simulink model "tools"  (R2019b)
settings: Solver=VariableStepAuto  StartTime=0.0  StopTime=10.0  RelTol=1e-3
undefined symbols (not defined in the file): pelvisPosition, pelvisVelocity, X, Y, Z
libraries: sm_lib x20, nesl_utility x13, ComponentLibrary x2
settings Model: Creator=hanli  LastModifiedBy=hanli

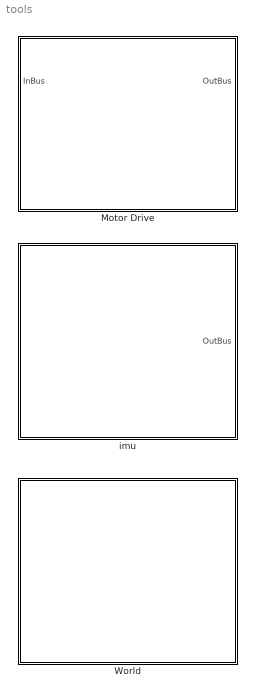
== system tools ==
  Motor Drive : Subsystem  AncestorBlock=ComponentLibrary/Simulation/Elmo Drive  mask{gearRatio=25, rotorInertia=0.000061, encoderResolution=2^13, peakTorque=4.5, peakSpeed=2900*(2*pi/60), initialPosition=0, initialVelocity=0}
      mask prompts: gearRatio "Gear Ratio:"; rotorInertia "Motor rotor inertia (kg*m^2):"; encoderResolution "Input Encoder Resolution (ticks/rev):"; peakTorque "Peak torque of motor (N*m):"; peakSpeed "Peak speed of motor (rad/s):"; initialPosition "Initial Position (rad):"; initialVelocity "Initial Velocity (rad/s):"
      mask Display: image('motor2.JPG'); % Use "Edit Image" on toolstrip to change.
  World : Subsystem  AncestorBlock=ComponentLibrary/Simulation/World
  imu : Subsystem  AncestorBlock=ComponentLibrary/Simulation/VectorNav  mask{preRotationMatrix=eye(3), postRotationMatrix=eye(3)}
      mask prompts: preRotationMatrix "Pre Rotation Matrix:"; postRotationMatrix "Post Rotation Matrix"
      mask Display: image('gx5-25.jpg'); % Use "Edit Image" on toolstrip to change.

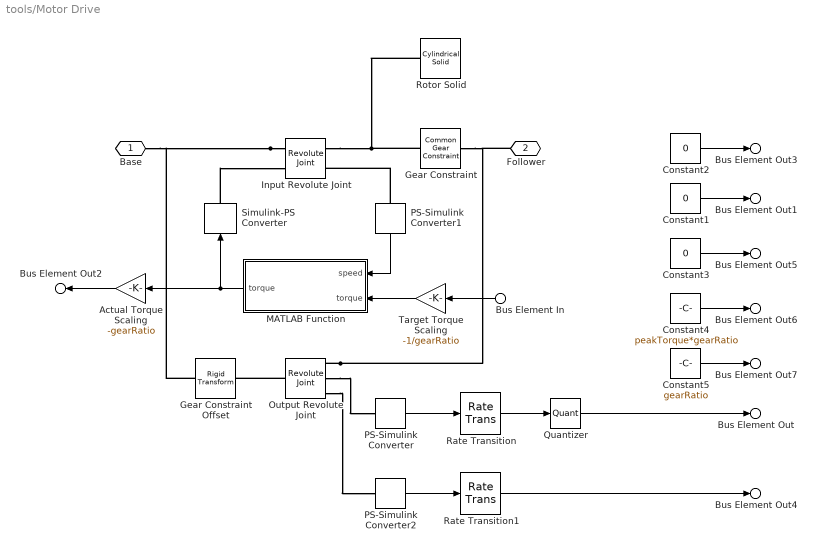
== system tools/Motor Drive ==
  Bus Element In : Inport  PortName=InBus  Element=torque
  Actual Torque Scaling : Gain  Gain=-gearRatio
  Constant1 : Constant  Value=0
  Constant2 : Constant  Value=0  OutDataTypeStr=uint16
  Constant3 : Constant  Value=0
  Constant4 : Constant  Value=peakTorque*gearRatio
  Constant5 : Constant  Value=gearRatio
  Gear Constraint : sm_lib/Gears and Couplings/Gears/Common Gear Constraint  GearType=External  SpecificationType=CenterDistanceRatio  CenterDistance=1e-6  CenterDistanceUnits=m  GearRatio=gearRatio  BaseGearRadius=10.0  BaseGearRadiusUnits=cm  FollGearRadius=10.0  FollGearRadiusUnits=cm  AssemblyGearRotation=Free
      settings: SourceProductName=Simscape Multibody  SourceProductBaseCode=MS
  Gear Constraint Offset : sm_lib/Frames and Transforms/Rigid Transform  TranslationMethod=StandardAxis  TranslationStandardOffset=1e-6  TranslationLengthUnit=m  TranslationStandardAxis=+Y  TranslationCartesianOffset=[0 0 0]  TranslationROffset=0  TranslationROffsetUnits=m  TranslationZOffset=0  TranslationZOffsetUnits=m  TranslationThetaOffset=0  TranslationThetaOffsetUnits=deg  RotationMethod=None  RotationAngleUnits=deg  RotationStandardAxis=+Z  RotationAngle=0.0  RotationArbitraryAxis=[0 0 1]  FollAlignAxisA=+X  BaseAlignAxisA=+Y  FollAlignAxisB=+Y  BaseAlignAxisB=+Z  RotationSequenceAxes=FollowerAxes  RotationSequence=XYX  RotationSequenceAngles=[0 0 0]  RotationSequenceAnglesUnits=deg  RotationMatrix=[1 0 0; 0 1 0; 0 0 1]
  Input Revolute Joint : sm_lib/Joints/Revolute Joint  JointMode=Normal  SenseConstraintForce=off  SenseConstraintForceX=off  SenseConstraintForceY=off  SenseConstraintForceZ=off  SenseConstraintTorque=off  SenseConstraintTorqueX=off  SenseConstraintTorqueY=off  SenseConstraintTorqueZ=off  SenseTotalForce=off  SenseTotalForceX=off  SenseTotalForceY=off  SenseTotalForceZ=off  SenseTotalTorque=off  SenseTotalTorqueX=off  SenseTotalTorqueY=off  SenseTotalTorqueZ=off  CompositeWrenchDir=FollowerOnBase  CompositeWrenchFrame=BaseFrame  EquilibriumPosition=0  EquilibriumPositionUnits=rad  SpringStiffness=0  SpringStiffnessUnits=N*m/rad  DampingCoefficient=0  DampingCoefficientUnits=N*m/(rad/s)  TorqueActuationMode=InputTorque  MotionActuationMode=ComputedMotion  SensePosition=off  SenseVelocity=on  SenseAcceleration=off  SenseTorqueForce=off  SenseLowerLimitTorqueForce=off  SenseUpperLimitTorqueForce=off  LowerLimitSpecify=off  LowerLimitBound=-90  LowerLimitBoundUnits=deg  LowerLimitStiffness=1e4  LowerLimitStiffnessUnits=N*m/deg  LowerLimitDamping=10  LowerLimitDampingUnits=N*m/(deg/s)  LowerLimitTransitionRegionWidth=0.1  LowerLimitTransitionRegionWidthUnits=deg  UpperLimitSpecify=off  UpperLimitBound=90  UpperLimitBoundUnits=deg  UpperLimitStiffness=1e4  UpperLimitStiffnessUnits=N*m/deg  UpperLimitDamping=10  UpperLimitDampingUnits=N*m/(deg/s)  UpperLimitTransitionRegionWidth=0.1  UpperLimitTransitionRegionWidthUnits=deg  PositionTargetSpecify=off  PositionTargetPriority=High  PositionTargetValue=0  PositionTargetValueUnits=deg  VelocityTargetSpecify=off  VelocityTargetPriority=High  VelocityTargetValue=0  VelocityTargetValueUnits=rad/s
  MATLAB Function : MATLAB Function  TreatAsAtomicUnit=on
  Output Revolute Joint : sm_lib/Joints/Revolute Joint  JointMode=Normal  SenseConstraintForce=off  SenseConstraintForceX=off  SenseConstraintForceY=off  SenseConstraintForceZ=off  SenseConstraintTorque=off  SenseConstraintTorqueX=off  SenseConstraintTorqueY=off  SenseConstraintTorqueZ=off  SenseTotalForce=off  SenseTotalForceX=off  SenseTotalForceY=off  SenseTotalForceZ=off  SenseTotalTorque=off  SenseTotalTorqueX=off  SenseTotalTorqueY=off  SenseTotalTorqueZ=off  CompositeWrenchDir=FollowerOnBase  CompositeWrenchFrame=BaseFrame  EquilibriumPosition=0  EquilibriumPositionUnits=rad  SpringStiffness=0  SpringStiffnessUnits=N*m/rad  DampingCoefficient=1  DampingCoefficientUnits=N*m/(rad/s)  TorqueActuationMode=NoTorque  MotionActuationMode=ComputedMotion  SensePosition=on  SenseVelocity=on  SenseAcceleration=off  SenseTorqueForce=off  SenseLowerLimitTorqueForce=off  SenseUpperLimitTorqueForce=off  LowerLimitSpecify=off  LowerLimitBound=-90  LowerLimitBoundUnits=deg  LowerLimitStiffness=1e4  LowerLimitStiffnessUnits=N*m/deg  LowerLimitDamping=10  LowerLimitDampingUnits=N*m/(deg/s)  LowerLimitTransitionRegionWidth=0.1  LowerLimitTransitionRegionWidthUnits=deg  UpperLimitSpecify=off  UpperLimitBound=90  UpperLimitBoundUnits=deg  UpperLimitStiffness=1e4  UpperLimitStiffnessUnits=N*m/deg  UpperLimitDamping=10  UpperLimitDampingUnits=N*m/(deg/s)  UpperLimitTransitionRegionWidth=0.1  UpperLimitTransitionRegionWidthUnits=deg  PositionTargetSpecify=on  PositionTargetPriority=High  PositionTargetValue=initialPosition  PositionTargetValueUnits=rad  VelocityTargetSpecify=on  VelocityTargetPriority=High  VelocityTargetValue=initialVelocity  VelocityTargetValueUnits=rad/s
  PS-Simulink Converter : nesl_utility/PS-Simulink Converter  PhysicalDomain=network_engine_domain  SubClassName=ps_output  LeftPortType=input  RightPortType=output  PseudoPeriodic=off  Frequencies=[]  Unit=rad  AffineConversion=off
  PS-Simulink Converter1 : nesl_utility/PS-Simulink Converter  PhysicalDomain=network_engine_domain  SubClassName=ps_output  LeftPortType=input  RightPortType=output  PseudoPeriodic=off  Frequencies=[]  Unit=rad/s  AffineConversion=off
  PS-Simulink Converter2 : nesl_utility/PS-Simulink Converter  PhysicalDomain=network_engine_domain  SubClassName=ps_output  LeftPortType=input  RightPortType=output  PseudoPeriodic=off  Frequencies=[]  Unit=rad/s  AffineConversion=off
  Quantizer : Quantizer  QuantizationInterval=(2*pi)/(encoderResolution*gearRatio)
  Rate Transition : RateTransition  Deterministic=off  InitialCondition=initialPosition  OutPortSampleTimeOpt=Inherit
  Rate Transition1 : RateTransition  Deterministic=off  InitialCondition=initialPosition  OutPortSampleTimeOpt=Inherit
  Rotor Solid : sm_lib/Body Elements/Cylindrical Solid  GraphicAmbientColor=[0.15 0.15 0.15 1.0]  BasedOnType=Density  CenterOfMass=[0; 0; 0]  CenterOfMassUnits=m  GraphicDiffuseColor=[0.5 0.5 0.5]  CylinderLength=1  CylinderLengthUnits=m  CylinderRadius=1  CylinderRadiusUnits=m  Density=1000  DensityUnits=kg/m^3  DoExposeReferenceFrame=on  GraphicEmissiveColor=[0.0 0.0 0.0 1.0]  ExportEntireGeometry=off  SerializedFrames=<Frames/>  MarkerShape=Sphere  MarkerSize=10  GraphicType=None  InertiaType=Custom  Mass=0  MassUnits=kg  MomentsOfInertia=[0; 0; rotorInertia]  MomentsOfInertiaUnits=kg*m^2  GraphicOpacity=1.0  ProductsOfInertia=[0; 0; 0]  ProductsOfInertiaUnits=kg*m^2  GraphicShininess=75  GraphicSpecularColor=[0.5 0.5 0.5 1.0]  GraphicVisPropType=SimpleVisualProperties
  Simulink-PS Converter : nesl_utility/Simulink-PS Converter  PhysicalDomain=network_engine_domain  SubClassName=ps_input  LeftPortType=input  RightPortType=output  PseudoPeriodic=off  Frequencies=[]  NoiseDistribution=none  NoiseParameters=[]  Unit=N*m  AffineConversion=off  FilteringAndDerivatives=zero  SimscapeFilterOrder=1  InputFilterTimeConstant=0.001  UdotUserProvided=1
  Target Torque Scaling : Gain  Gain=-1/gearRatio
  Base : PMIOPort  Side=Left
  Follower : PMIOPort  Port=2  Side=Right
  Bus Element Out3 : Outport  VectorParamsAs1DForOutWhenUnconnected=off  PortName=OutBus  Element=statusWord
  Bus Element Out : Outport  VectorParamsAs1DForOutWhenUnconnected=off  PortName=OutBus  Element=position
  Bus Element Out4 : Outport  VectorParamsAs1DForOutWhenUnconnected=off  PortName=OutBus  Element=velocity
  Bus Element Out2 : Outport  VectorParamsAs1DForOutWhenUnconnected=off  PortName=OutBus  Element=torque
  Bus Element Out1 : Outport  VectorParamsAs1DForOutWhenUnconnected=off  PortName=OutBus  Element=driveTemperature
  Bus Element Out5 : Outport  VectorParamsAs1DForOutWhenUnconnected=off  PortName=OutBus  Element=dcLinkVoltage
  Bus Element Out6 : Outport  VectorParamsAs1DForOutWhenUnconnected=off  PortName=OutBus  Element=torqueLimit
  Bus Element Out7 : Outport  VectorParamsAs1DForOutWhenUnconnected=off  PortName=OutBus  Element=gearRatio
  wires:
  PS-Simulink Converter2/1 -> Rate Transition1/1
  Rate Transition1/1 -> Bus Element Out4/1
  Constant5/1 -> Bus Element Out7/1
  Actual Torque Scaling/1 -> Bus Element Out2/1
  Constant4/1 -> Bus Element Out6/1
  Constant3/1 -> Bus Element Out5/1
  Constant1/1 -> Bus Element Out1/1
  Constant2/1 -> Bus Element Out3/1
  Target Torque Scaling/1 -> MATLAB Function/2("torque ")
  PS-Simulink Converter1/1 -> MATLAB Function/1(speed)
  MATLAB Function/1(torque) -> Simulink-PS Converter/1, Actual Torque Scaling/1
  Bus Element In/1 -> Target Torque Scaling/1
  Quantizer/1 -> Bus Element Out/1
  PS-Simulink Converter/1 -> Rate Transition/1
  Rate Transition/1 -> Quantizer/1
  connections:
  Output Revolute Joint/RConn3 -- PS-Simulink Converter2/LConn1
  Input Revolute Joint/LConn1 -- Base/RConn1 -- Gear Constraint Offset/LConn1
  Simulink-PS Converter/RConn1 -- Input Revolute Joint/LConn2
  PS-Simulink Converter1/LConn1 -- Input Revolute Joint/RConn2
  Rotor Solid/RConn1 -- Gear Constraint/LConn1 -- Input Revolute Joint/RConn1
  Output Revolute Joint/RConn1 -- Follower/RConn1 -- Gear Constraint/RConn1
  Output Revolute Joint/LConn1 -- Gear Constraint Offset/RConn1
  Output Revolute Joint/RConn2 -- PS-Simulink Converter/LConn1

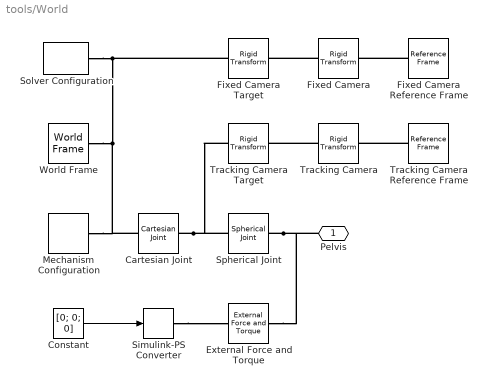
== system tools/World ==
  Cartesian Joint : sm_lib/Joints/Cartesian Joint  JointMode=Normal  SenseConstraintForce=off  SenseConstraintForceX=off  SenseConstraintForceY=off  SenseConstraintForceZ=off  SenseConstraintTorque=off  SenseConstraintTorqueX=off  SenseConstraintTorqueY=off  SenseConstraintTorqueZ=off  SenseTotalForce=off  SenseTotalForceX=off  SenseTotalForceY=off  SenseTotalForceZ=off  SenseTotalTorque=off  SenseTotalTorqueX=off  SenseTotalTorqueY=off  SenseTotalTorqueZ=off  CompositeWrenchDir=FollowerOnBase  CompositeWrenchFrame=BaseFrame  PxEquilibriumPosition=0  PxEquilibriumPositionUnits=m  PxSpringStiffness=0  PxSpringStiffnessUnits=N/m  PxDampingCoefficient=0  PxDampingCoefficientUnits=N/(m/s)  PxTorqueActuationMode=NoTorque  PxMotionActuationMode=ComputedMotion  PxSensePosition=off  PxSenseVelocity=off  PxSenseAcceleration=off  PxSenseTorqueForce=off  PxSenseLowerLimitTorqueForce=off  PxSenseUpperLimitTorqueForce=off  PxLowerLimitSpecify=off  PxLowerLimitBound=-1  PxLowerLimitBoundUnits=m  PxLowerLimitStiffness=1e6  PxLowerLimitStiffnessUnits=N/m  PxLowerLimitDamping=1e3  PxLowerLimitDampingUnits=N/(m/s)  PxLowerLimitTransitionRegionWidth=1e-4  PxLowerLimitTransitionRegionWidthUnits=m  PxUpperLimitSpecify=off  PxUpperLimitBound=1  PxUpperLimitBoundUnits=m  PxUpperLimitStiffness=1e6  PxUpperLimitStiffnessUnits=N/m  PxUpperLimitDamping=1e3  PxUpperLimitDampingUnits=N/(m/s)  PxUpperLimitTransitionRegionWidth=1e-4  PxUpperLimitTransitionRegionWidthUnits=m  PxPositionTargetSpecify=on  PxPositionTargetPriority=High  PxPositionTargetValue=pelvisPosition(1)  PxPositionTargetValueUnits=m  PxVelocityTargetSpecify=on  PxVelocityTargetPriority=High  PxVelocityTargetValue=pelvisVelocity(1)  PxVelocityTargetValueUnits=m/s  PyEquilibriumPosition=0  PyEquilibriumPositionUnits=m  PySpringStiffness=0  PySpringStiffnessUnits=N/m  PyDampingCoefficient=0  PyDampingCoefficientUnits=N/(m/s)  PyTorqueActuationMode=NoTorque  PyMotionActuationMode=ComputedMotion  PySensePosition=off  PySenseVelocity=off  PySenseAcceleration=off  PySenseTorqueForce=off  PySenseLowerLimitTorqueForce=off  PySenseUpperLimitTorqueForce=off  PyLowerLimitSpecify=off  PyLowerLimitBound=-1  PyLowerLimitBoundUnits=m  PyLowerLimitStiffness=1e6  PyLowerLimitStiffnessUnits=N/m  PyLowerLimitDamping=1e3  PyLowerLimitDampingUnits=N/(m/s)  PyLowerLimitTransitionRegionWidth=1e-4  PyLowerLimitTransitionRegionWidthUnits=m  PyUpperLimitSpecify=off  PyUpperLimitBound=1  PyUpperLimitBoundUnits=m  PyUpperLimitStiffness=1e6  PyUpperLimitStiffnessUnits=N/m  PyUpperLimitDamping=1e3  PyUpperLimitDampingUnits=N/(m/s)  PyUpperLimitTransitionRegionWidth=1e-4  PyUpperLimitTransitionRegionWidthUnits=m  PyPositionTargetSpecify=on  PyPositionTargetPriority=High  PyPositionTargetValue=pelvisPosition(2)  PyPositionTargetValueUnits=m  PyVelocityTargetSpecify=on  PyVelocityTargetPriority=High  PyVelocityTargetValue=pelvisVelocity(2)  PyVelocityTargetValueUnits=m/s  PzEquilibriumPosition=0  PzEquilibriumPositionUnits=m  PzSpringStiffness=0  PzSpringStiffnessUnits=N/m  PzDampingCoefficient=0  PzDampingCoefficientUnits=N/(m/s)  PzTorqueActuationMode=NoTorque  PzMotionActuationMode=ComputedMotion  PzSensePosition=off  PzSenseVelocity=off  PzSenseAcceleration=off  PzSenseTorqueForce=off  PzSenseLowerLimitTorqueForce=off  PzSenseUpperLimitTorqueForce=off  PzLowerLimitSpecify=off  PzLowerLimitBound=-1  PzLowerLimitBoundUnits=m  PzLowerLimitStiffness=1e6  PzLowerLimitStiffnessUnits=N/m  PzLowerLimitDamping=1e3  PzLowerLimitDampingUnits=N/(m/s)  PzLowerLimitTransitionRegionWidth=1e-4  PzLowerLimitTransitionRegionWidthUnits=m  PzUpperLimitSpecify=off  PzUpperLimitBound=1  PzUpperLimitBoundUnits=m  PzUpperLimitStiffness=1e6  PzUpperLimitStiffnessUnits=N/m  PzUpperLimitDamping=1e3  PzUpperLimitDampingUnits=N/(m/s)  PzUpperLimitTransitionRegionWidth=1e-4  PzUpperLimitTransitionRegionWidthUnits=m  PzPositionTargetSpecify=on  PzPositionTargetPriority=High  PzPositionTargetValue=pelvisPosition(3)  PzPositionTargetValueUnits=m  PzVelocityTargetSpecify=on  PzVelocityTargetPriority=High  PzVelocityTargetValue=pelvisVelocity(3)  PzVelocityTargetValueUnits=m/s
  Constant : Constant  Value=[0; 0; 0]
  External Force and Torque : sm_lib/Forces and Torques/External Force and Torque  ForceResolutionFrame=World  EnableForceX=off  EnableForceY=off  EnableForceZ=off  EnableForce=on  TorqueResolutionFrame=AttachedFrame  EnableTorqueX=off  EnableTorqueY=off  EnableTorqueZ=off  EnableTorque=off
  Fixed Camera : sm_lib/Frames and Transforms/Rigid Transform  TranslationMethod=Cartesian  TranslationStandardOffset=0  TranslationLengthUnit=m  TranslationStandardAxis=+Z  TranslationCartesianOffset=[1.5 -1.5 0.5]  TranslationROffset=0  TranslationROffsetUnits=m  TranslationZOffset=0  TranslationZOffsetUnits=m  TranslationThetaOffset=0  TranslationThetaOffsetUnits=deg  RotationMethod=None  RotationAngleUnits=deg  RotationStandardAxis=+Z  RotationAngle=0.0  RotationArbitraryAxis=[0 0 1]  FollAlignAxisA=+X  BaseAlignAxisA=+Y  FollAlignAxisB=+Y  BaseAlignAxisB=+Z  RotationSequenceAxes=FollowerAxes  RotationSequence=XYX  RotationSequenceAngles=[0 0 0]  RotationSequenceAnglesUnits=deg  RotationMatrix=[1 0 0; 0 1 0; 0 0 1]
  Fixed Camera Target : sm_lib/Frames and Transforms/Rigid Transform  TranslationMethod=Cartesian  TranslationStandardOffset=0  TranslationLengthUnit=m  TranslationStandardAxis=+Z  TranslationCartesianOffset=[0 0 0.5]  TranslationROffset=0  TranslationROffsetUnits=m  TranslationZOffset=0  TranslationZOffsetUnits=m  TranslationThetaOffset=0  TranslationThetaOffsetUnits=deg  RotationMethod=None  RotationAngleUnits=deg  RotationStandardAxis=+Z  RotationAngle=0.0  RotationArbitraryAxis=[0 0 1]  FollAlignAxisA=+X  BaseAlignAxisA=+Y  FollAlignAxisB=+Y  BaseAlignAxisB=+Z  RotationSequenceAxes=FollowerAxes  RotationSequence=XYX  RotationSequenceAngles=[0 0 0]  RotationSequenceAnglesUnits=deg  RotationMatrix=[1 0 0; 0 1 0; 0 0 1]
  Fixed Camera Reference Frame : sm_lib/Frames and Transforms/Reference Frame
  Mechanism Configuration : sm_lib/Utilities/Mechanism Configuration  UniformGravity=Constant  GravityVector=[0 0 -9.80665]  GravityUnits=m/s^2  LinearizationDelta=0.001
  Simulink-PS Converter : nesl_utility/Simulink-PS Converter  PhysicalDomain=network_engine_domain  SubClassName=ps_input  LeftPortType=input  RightPortType=output  PseudoPeriodic=off  Frequencies=[]  NoiseDistribution=none  NoiseParameters=[]  Unit=1  AffineConversion=off  FilteringAndDerivatives=provide  SimscapeFilterOrder=1  InputFilterTimeConstant=0.001  UdotUserProvided=0
  Solver Configuration : nesl_utility/Solver Configuration  PhysicalDomain=network_engine_domain  SubClassName=solver  LeftPortType=input  RightPortType=generic  Tones=[]  Harmonics=[]  SimulateNoise=off  Profile=off  UseLocalSampling=off  EnableSwitchedLinearOptims=on  FrequencyDomain=off  UseCCode=off  RelTol=0.001  AbsTol=1e-06  MinStep=1e-09  ToWorkspace=off  RevertToSquareIcSolve=off  NumHomotopyIterations=100  PhasorMode=off  PhasorModeNumHarmonics=1  DoDC=off  ResidualTolerance=1e-09  UseLocalSolver=off  LocalSolverChoice=NE_BACKWARD_EULER_ADVANCER  LocalSolverSampleTime=0.001  DoFixedCost=off  MaxNonlinIter=3  MaxModeIter=2  LinearAlgebra=Sparse  EquationFormulation=NE_TIME_EF  DelaysMemoryBudget=1024  AutomaticFiltering=on  FilteringTimeConstant=0.001  PartitionStorageMethod=AS_NEEDED  PartitionMemoryBudget=1024  PartitionMethod=FAST
  Spherical Joint : sm_lib/Joints/Spherical Joint  JointMode=Normal  SenseConstraintForce=off  SenseConstraintForceX=off  SenseConstraintForceY=off  SenseConstraintForceZ=off  SenseConstraintTorque=off  SenseConstraintTorqueX=off  SenseConstraintTorqueY=off  SenseConstraintTorqueZ=off  SenseTotalForce=off  SenseTotalForceX=off  SenseTotalForceY=off  SenseTotalForceZ=off  SenseTotalTorque=off  SenseTotalTorqueX=off  SenseTotalTorqueY=off  SenseTotalTorqueZ=off  CompositeWrenchDir=FollowerOnBase  CompositeWrenchFrame=BaseFrame  DefPosRotationMethod=None  DefPosRotationAngleUnits=deg  DefPosRotationStandardAxis=+Z  DefPosRotationAngle=0.0  DefPosRotationArbitraryAxis=[0 0 1]  DefPosFollAlignAxisA=+X  DefPosBaseAlignAxisA=+Y  DefPosFollAlignAxisB=+Y  DefPosBaseAlignAxisB=+Z  DefPosRotationSequenceAxes=FollowerAxes  DefPosRotationSequence=XYX  DefPosRotationSequenceAngles=[0 0 0]  DefPosRotationSequenceAnglesUnits=deg  DefPosRotationMatrix=[1 0 0; 0 1 0; 0 0 1]  EqPosRotationMethod=None  EqPosRotationAngleUnits=deg  EqPosRotationStandardAxis=+Z  EqPosRotationAngle=0.0  EqPosRotationArbitraryAxis=[0 0 1]  EqPosFollAlignAxisA=+X  EqPosBaseAlignAxisA=+Y  EqPosFollAlignAxisB=+Y  EqPosBaseAlignAxisB=+Z  EqPosRotationSequenceAxes=FollowerAxes  EqPosRotationSequence=XYX  EqPosRotationSequenceAngles=[0 0 0]  EqPosRotationSequenceAnglesUnits=deg  EqPosRotationMatrix=[1 0 0; 0 1 0; 0 0 1]  SpringStiffness=0  SpringStiffnessUnits=N*m/deg  DampingCoefficient=0  DampingCoefficientUnits=N*m/(deg/s)  ActuateTorqueX=off  ActuateTorqueY=off  ActuateTorqueZ=off  ActuateTorque=off  TorqueActuationMode=NoTorque  MotionActuationMode=ComputedMotion  ActuationFrame=BaseFrame  SensePosition=off  SenseVelocityX=off  SenseVelocityY=off  SenseVelocityZ=off  SenseVelocity=off  SenseAccelerationX=off  SenseAccelerationY=off  SenseAccelerationZ=off  SenseAcceleration=off  SenseTorqueX=off  SenseTorqueY=off  SenseTorqueZ=off  SenseTorqueForce=off  SenseLowerLimitTorqueMag=off  SenseUpperLimitTorqueMag=off  SensingFrame=BaseFrame  LowerLimitSpecify=off  LowerLimitBound=15  LowerLimitBoundUnits=deg  LowerLimitStiffness=1e4  LowerLimitStiffnessUnits=N*m/deg  LowerLimitDamping=10  LowerLimitDampingUnits=N*m/(deg/s)  LowerLimitTransitionRegionWidth=0.1  LowerLimitTransitionRegionWidthUnits=deg  UpperLimitSpecify=off  UpperLimitBound=45  UpperLimitBoundUnits=deg  UpperLimitStiffness=1e4  UpperLimitStiffnessUnits=N*m/deg  UpperLimitDamping=10  UpperLimitDampingUnits=N*m/(deg/s)  UpperLimitTransitionRegionWidth=0.1  UpperLimitTransitionRegionWidthUnits=deg  PositionTargetRotationMethod=RotationMatrix  PositionTargetRotationAngleUnits=deg  PositionTargetRotationStandardAxis=+Z  PositionTargetRotationAngle=0.0  PositionTargetRotationArbitraryAxis=[0 0 1]  PositionTargetFollAlignAxisA=+X  PositionTargetBaseAlignAxisA=+Y  PositionTargetFollAlignAxisB=+Y  PositionTargetBaseAlignAxisB=+Z  PositionTargetRotationSequenceAxes=FollowerAxes  PositionTargetRotationSequence=XYX  PositionTargetRotationSequenceAngles=[0 0 0]  PositionTargetRotationSequenceAnglesUnits=deg  PositionTargetRotationMatrix=pelvisRotation  PositionTargetSpecify=on  PositionTargetPriority=High  VelocityTargetValue=pelvisAngularVelocity  VelocityTargetValueUnits=rad/s  VelocityTargetSpecify=on  VelocityTargetPriority=High  VelocityTargetInFollowerFrame=on
  Tracking Camera : sm_lib/Frames and Transforms/Rigid Transform  TranslationMethod=Cartesian  TranslationStandardOffset=0  TranslationLengthUnit=m  TranslationStandardAxis=+Z  TranslationCartesianOffset=[1.5 -1.5 0.5]  TranslationROffset=0  TranslationROffsetUnits=m  TranslationZOffset=0  TranslationZOffsetUnits=m  TranslationThetaOffset=0  TranslationThetaOffsetUnits=deg  RotationMethod=None  RotationAngleUnits=deg  RotationStandardAxis=+Z  RotationAngle=0.0  RotationArbitraryAxis=[0 0 1]  FollAlignAxisA=+X  BaseAlignAxisA=+Y  FollAlignAxisB=+Y  BaseAlignAxisB=+Z  RotationSequenceAxes=FollowerAxes  RotationSequence=XYX  RotationSequenceAngles=[0 0 0]  RotationSequenceAnglesUnits=deg  RotationMatrix=[1 0 0; 0 1 0; 0 0 1]
  Tracking Camera Target : sm_lib/Frames and Transforms/Rigid Transform  TranslationMethod=Cartesian  TranslationStandardOffset=0  TranslationLengthUnit=m  TranslationStandardAxis=+Z  TranslationCartesianOffset=[0 0 -0.5]  TranslationROffset=0  TranslationROffsetUnits=m  TranslationZOffset=0  TranslationZOffsetUnits=m  TranslationThetaOffset=0  TranslationThetaOffsetUnits=deg  RotationMethod=None  RotationAngleUnits=deg  RotationStandardAxis=+Z  RotationAngle=0.0  RotationArbitraryAxis=[0 0 1]  FollAlignAxisA=+X  BaseAlignAxisA=+Y  FollAlignAxisB=+Y  BaseAlignAxisB=+Z  RotationSequenceAxes=FollowerAxes  RotationSequence=XYX  RotationSequenceAngles=[0 0 0]  RotationSequenceAnglesUnits=deg  RotationMatrix=[1 0 0; 0 1 0; 0 0 1]
  Tracking Camera Reference Frame : sm_lib/Frames and Transforms/Reference Frame
  World Frame : sm_lib/Frames and Transforms/World Frame
  Pelvis : PMIOPort  Side=Right
  wires:
  Constant/1 -> Simulink-PS Converter/1
  connections:
  Simulink-PS Converter/RConn1 -- External Force and Torque/LConn1
  Fixed Camera/LConn1 -- Fixed Camera Target/RConn1
  Fixed Camera Reference Frame/RConn1 -- Fixed Camera/RConn1
  Tracking Camera/LConn1 -- Tracking Camera Target/RConn1
  Tracking Camera Reference Frame/RConn1 -- Tracking Camera/RConn1
  Fixed Camera Target/LConn1 -- Solver Configuration/RConn1 -- Cartesian Joint/LConn1 -- Mechanism Configuration/RConn1 -- World Frame/RConn1
  Spherical Joint/RConn1 -- External Force and Torque/RConn1 -- Pelvis/RConn1
  Cartesian Joint/RConn1 -- Tracking Camera Target/LConn1 -- Spherical Joint/LConn1

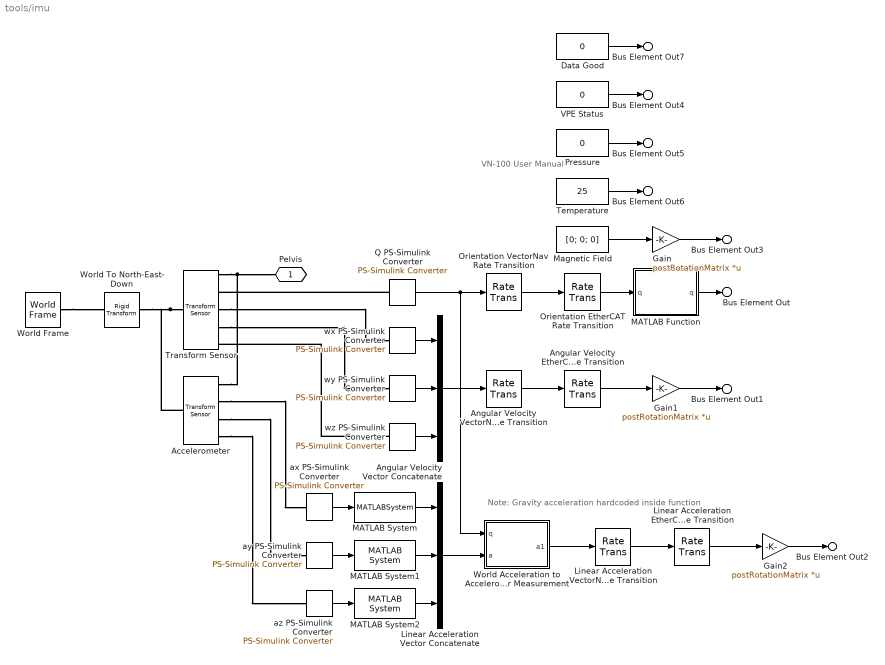
== system tools/imu ==
  note: VN-100 User Manual
  note: Note: Gravity acceleration hardcoded inside function
  Accelerometer : sm_lib/Frames and Transforms/Transform Sensor  MeasurementFrame=Base  SenseAngle=off  SenseAxis=off  SenseAngle1=off  SenseAngle2=off  SenseAngle3=off  SenseQ=off  SenseR=off  SenseOmegaX=off  SenseOmegaY=off  SenseOmegaZ=off  SenseOmega1=off  SenseOmega2=off  SenseOmega3=off  SenseQDot=off  SenseRDot=off  SenseAlphaX=off  SenseAlphaY=off  SenseAlphaZ=off  SenseAlpha1=off  SenseAlpha2=off  SenseAlpha3=off  SenseQDDot=off  SenseRDDot=off  SenseX=off  SenseY=off  SenseZ=off  SenseRad=off  SenseAzim=off  SenseDist=off  SenseInc=off  SenseXDot=off  SenseYDot=off  SenseZDot=off  SenseRadDot=off  SenseAzimDot=off  SenseDistDot=off  SenseIncDot=off  SenseXDDot=on  SenseYDDot=on  SenseZDDot=on  SenseRadDDot=off  SenseAzimDDot=off  SenseDistDDot=off  SenseIncDDot=off
  Angular Velocity EtherCAT Rate Transition : RateTransition  Deterministic=off  OutPortSampleTimeOpt=Inherit
  Angular Velocity Vector Concatenate : Concatenate  NumInputs=3
  Angular Velocity VectorNav Rate Transition : RateTransition  Deterministic=off  OutPortSampleTime=VectorNavModule.sampleTime
  Data Good : Constant  Value=0  OutDataTypeStr=boolean
  Gain : Gain  Gain=postRotationMatrix  Multiplication=Matrix(K*u)
  Gain1 : Gain  Gain=postRotationMatrix  Multiplication=Matrix(K*u)
  Gain2 : Gain  Gain=postRotationMatrix  Multiplication=Matrix(K*u)
  Linear Acceleration EtherCAT Rate Transition : RateTransition  Deterministic=off  InitialCondition=[0; 0; 0]  OutPortSampleTimeOpt=Inherit
  Linear Acceleration Vector Concatenate : Concatenate  NumInputs=3
  Linear Acceleration VectorNav Rate Transition : RateTransition  Deterministic=off  InitialCondition=[0; 0; 0]  OutPortSampleTime=VectorNavModule.sampleTime
  MATLAB Function : MATLAB Function  TreatAsAtomicUnit=on
  MATLAB System : MATLABSystem  System=FilterSystem  a=[1 -0.8]  b=0.2  SimulateUsing=Code generation
      mask Type: FilterSystem
      mask Display: disp('Filter');
  MATLAB System1 : ComponentLibrary/Simulation/VectorNav/MATLAB System  a=[1 -0.8]  b=0.2  SimulateUsing=Code generation
  MATLAB System2 : ComponentLibrary/Simulation/VectorNav/MATLAB System  a=[1 -0.8]  b=0.2  SimulateUsing=Code generation
  Magnetic Field : Constant  Value=[0; 0; 0]
  Orientation EtherCAT Rate Transition : RateTransition  Deterministic=off  InitialCondition=[0; 0; 0; 1]  OutPortSampleTimeOpt=Inherit
  Orientation VectorNav Rate Transition : RateTransition  Deterministic=off  InitialCondition=[0; 0; 0; 1]  OutPortSampleTime=VectorNavModule.sampleTime
  Pressure : Constant  Value=0
  Q PS-Simulink Converter : nesl_utility/PS-Simulink Converter  PhysicalDomain=network_engine_domain  SubClassName=ps_output  LeftPortType=input  RightPortType=output  PseudoPeriodic=off  Frequencies=[]  Unit=1  AffineConversion=off
  Temperature : Constant  Value=25
  Transform Sensor : sm_lib/Frames and Transforms/Transform Sensor  MeasurementFrame=Follower  SenseAngle=off  SenseAxis=off  SenseAngle1=off  SenseAngle2=off  SenseAngle3=off  SenseQ=on  SenseR=off  SenseOmegaX=on  SenseOmegaY=on  SenseOmegaZ=on  SenseOmega1=off  SenseOmega2=off  SenseOmega3=off  SenseQDot=off  SenseRDot=off  SenseAlphaX=off  SenseAlphaY=off  SenseAlphaZ=off  SenseAlpha1=off  SenseAlpha2=off  SenseAlpha3=off  SenseQDDot=off  SenseRDDot=off  SenseX=off  SenseY=off  SenseZ=off  SenseRad=off  SenseAzim=off  SenseDist=off  SenseInc=off  SenseXDot=off  SenseYDot=off  SenseZDot=off  SenseRadDot=off  SenseAzimDot=off  SenseDistDot=off  SenseIncDot=off  SenseXDDot=off  SenseYDDot=off  SenseZDDot=off  SenseRadDDot=off  SenseAzimDDot=off  SenseDistDDot=off  SenseIncDDot=off
  VPE Status : Constant  Value=0  OutDataTypeStr=uint16
  World Acceleration to Accelerometer Measurement : MATLAB Function  TreatAsAtomicUnit=on
  World Frame : sm_lib/Frames and Transforms/World Frame
  World To North-East-Down : sm_lib/Frames and Transforms/Rigid Transform  TranslationMethod=None  TranslationStandardOffset=0  TranslationLengthUnit=m  TranslationStandardAxis=+Z  TranslationCartesianOffset=[0 0 0]  TranslationROffset=0  TranslationROffsetUnits=m  TranslationZOffset=0  TranslationZOffsetUnits=m  TranslationThetaOffset=0  TranslationThetaOffsetUnits=deg  RotationMethod=StandardAxis  RotationAngleUnits=deg  RotationStandardAxis=+X  RotationAngle=180  RotationArbitraryAxis=[0 0 1]  FollAlignAxisA=+X  BaseAlignAxisA=+Y  FollAlignAxisB=+Y  BaseAlignAxisB=+Z  RotationSequenceAxes=FollowerAxes  RotationSequence=XYX  RotationSequenceAngles=[0 0 0]  RotationSequenceAnglesUnits=deg  RotationMatrix=[1 0 0; 0 1 0; 0 0 1]
  ax PS-Simulink Converter : nesl_utility/PS-Simulink Converter  PhysicalDomain=network_engine_domain  SubClassName=ps_output  LeftPortType=input  RightPortType=output  PseudoPeriodic=off  Frequencies=[]  Unit=m/s/s  AffineConversion=off
  ay PS-Simulink Converter : nesl_utility/PS-Simulink Converter  PhysicalDomain=network_engine_domain  SubClassName=ps_output  LeftPortType=input  RightPortType=output  PseudoPeriodic=off  Frequencies=[]  Unit=m/s/s  AffineConversion=off
  az PS-Simulink Converter : nesl_utility/PS-Simulink Converter  PhysicalDomain=network_engine_domain  SubClassName=ps_output  LeftPortType=input  RightPortType=output  PseudoPeriodic=off  Frequencies=[]  Unit=m/s/s  AffineConversion=off
  wx PS-Simulink Converter : nesl_utility/PS-Simulink Converter  PhysicalDomain=network_engine_domain  SubClassName=ps_output  LeftPortType=input  RightPortType=output  PseudoPeriodic=off  Frequencies=[]  Unit=1  AffineConversion=off
  wy PS-Simulink Converter : nesl_utility/PS-Simulink Converter  PhysicalDomain=network_engine_domain  SubClassName=ps_output  LeftPortType=input  RightPortType=output  PseudoPeriodic=off  Frequencies=[]  Unit=1  AffineConversion=off
  wz PS-Simulink Converter : nesl_utility/PS-Simulink Converter  PhysicalDomain=network_engine_domain  SubClassName=ps_output  LeftPortType=input  RightPortType=output  PseudoPeriodic=off  Frequencies=[]  Unit=1  AffineConversion=off
  Pelvis : PMIOPort  Side=Left
  Bus Element Out7 : Outport  VectorParamsAs1DForOutWhenUnconnected=off  PortName=OutBus  Element=dataGood
  Bus Element Out4 : Outport  VectorParamsAs1DForOutWhenUnconnected=off  PortName=OutBus  Element=vpeStatus
  Bus Element Out5 : Outport  VectorParamsAs1DForOutWhenUnconnected=off  PortName=OutBus  Element=pressure
  Bus Element Out6 : Outport  VectorParamsAs1DForOutWhenUnconnected=off  PortName=OutBus  Element=temperature
  Bus Element Out3 : Outport  VectorParamsAs1DForOutWhenUnconnected=off  PortName=OutBus  Element=magneticField
  Bus Element Out1 : Outport  VectorParamsAs1DForOutWhenUnconnected=off  PortName=OutBus  Element=angularVelocity
  Bus Element Out2 : Outport  VectorParamsAs1DForOutWhenUnconnected=off  PortName=OutBus  Element=linearAcceleration
  Bus Element Out : Outport  VectorParamsAs1DForOutWhenUnconnected=off  PortName=OutBus  Element=orientation
  wires:
  Linear Acceleration Vector Concatenate/1 -> World Acceleration to Accelerometer Measurement/2(a)
  World Acceleration to Accelerometer Measurement/1(a1) -> Linear Acceleration VectorNav Rate Transition/1
  Gain2/1 -> Bus Element Out2/1
  MATLAB System2/1 -> Linear Acceleration Vector Concatenate/3
  MATLAB System1/1 -> Linear Acceleration Vector Concatenate/2
  MATLAB System/1 -> Linear Acceleration Vector Concatenate/1
  MATLAB Function/1(q) -> Bus Element Out/1
  Gain1/1 -> Bus Element Out1/1
  Gain/1 -> Bus Element Out3/1
  Pressure/1 -> Bus Element Out5/1
  Angular Velocity Vector Concatenate/1 -> Angular Velocity VectorNav Rate Transition/1
  Magnetic Field/1 -> Gain/1
  ay PS-Simulink Converter/1 -> MATLAB System1/1
  Data Good/1 -> Bus Element Out7/1
  Linear Acceleration VectorNav Rate Transition/1 -> Linear Acceleration EtherCAT Rate Transition/1
  Linear Acceleration EtherCAT Rate Transition/1 -> Gain2/1
  Orientation VectorNav Rate Transition/1 -> Orientation EtherCAT Rate Transition/1
  Angular Velocity EtherCAT Rate Transition/1 -> Gain1/1
  wy PS-Simulink Converter/1 -> Angular Velocity Vector Concatenate/2
  Temperature/1 -> Bus Element Out6/1
  Q PS-Simulink Converter/1 -> Orientation VectorNav Rate Transition/1, World Acceleration to Accelerometer Measurement/1(q)
  Orientation EtherCAT Rate Transition/1 -> MATLAB Function/1("q ")
  VPE Status/1 -> Bus Element Out4/1
  ax PS-Simulink Converter/1 -> MATLAB System/1
  wx PS-Simulink Converter/1 -> Angular Velocity Vector Concatenate/1
  az PS-Simulink Converter/1 -> MATLAB System2/1
  wz PS-Simulink Converter/1 -> Angular Velocity Vector Concatenate/3
  Angular Velocity VectorNav Rate Transition/1 -> Angular Velocity EtherCAT Rate Transition/1
  connections:
  wz PS-Simulink Converter/LConn1 -- Transform Sensor/RConn5
  Transform Sensor/RConn3 -- wx PS-Simulink Converter/LConn1
  Accelerometer/RConn4 -- az PS-Simulink Converter/LConn1
  Accelerometer/RConn1 -- Pelvis/RConn1 -- Transform Sensor/RConn1
  Accelerometer/RConn2 -- ax PS-Simulink Converter/LConn1
  Q PS-Simulink Converter/LConn1 -- Transform Sensor/RConn2
  World Frame/RConn1 -- World To North-East-Down/LConn1
  Accelerometer/RConn3 -- ay PS-Simulink Converter/LConn1
  Transform Sensor/LConn1 -- Accelerometer/LConn1 -- World To North-East-Down/RConn1
  Transform Sensor/RConn4 -- wy PS-Simulink Converter/LConn1

== matlab function tools/Motor Drive/MATLAB Function ==
  data: speed input; torque output; torque input; peakTorque parameter; peakSpeed parameter
function torque = fcn(speed, torque, peakTorque, peakSpeed) %#codegen

  % Cap the velocity at the specified limits to avoid extrapolation
  speed = median([-peakSpeed, speed, peakSpeed]);

  % Linear interpolation of speed-torque curve
  torqueLimit = interp1(...
    [0, 0.5*peakSpeed, peakSpeed], ...
    [peakTorque, peakTorque, 0], ...
    abs(speed));

  % Cap the torque command at the specified imits
  torque = median([-torqueLimit, torque, torqueLimit]);
end % fcn

== matlab function tools/imu/MATLAB Function ==
  data: q input; q output; preRotationMatrix parameter; postRotationMatrix parameter
function q = fcn(q, preRotationMatrix, postRotationMatrix)
  % Construct constant rotation matrix objects
  R0 = coder.const(Rotation3d(preRotationMatrix));
  R2 = coder.const(Rotation3d(postRotationMatrix));
  
  % Convert rotation matrices into constant quaternion objects
  Q0 = coder.const(R0.getQuaternion);
  Q2 = coder.const(R2.getQuaternion);
  
  % Apply pre and post rotations
  Q1 = Q0*Quaternion(q)*Q2;
  
  % Convert quaternion object to double
  q = Q1.getValue;
end % fcn

== matlab function tools/imu/World Acceleration to Accelerometer Measurement ==
  data: q input; a1 output; a input
function a1 = fcn(q, a)
  % Construct quaternion object
  Q = Quaternion(q);
  
  % Add world gravity acceleration to body acceleration
  a1 = Q.getRotation.getValue'*(a + [0; 0; -9.806]);
end % fcn
